simulink model "Counter_Down"  (R2016b)
settings: Solver=VariableStepAuto  StartTime=0.0  StopTime=10.0  RelTol=1e-3
settings Model: Creator=Saher Ghanem  LastModifiedBy=Saher Ghanem

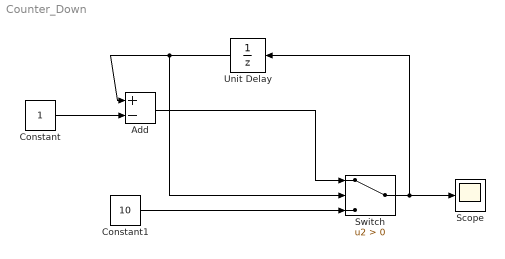
== system Counter_Down ==
  Add : Sum  Inputs=+-
  Constant : Constant
  Constant1 : Constant  Value=10
  Scope : Scope
  Switch : Switch  Criteria=u2 > Threshold
  Unit Delay : UnitDelay  SampleTime=-1
  wires:
  Constant/1 -> Add/2
  Switch/1 -> Scope/1, Unit Delay/1
  Constant1/1 -> Switch/3
  Add/1 -> Switch/1
  Unit Delay/1 -> Switch/2, Add/1
